simulink model "Projet_Controle_Trajectoire_drone"  (R2024a)
settings: Solver=ode4  StartTime=0.0  StopTime=Tfinsim  FixedStep=Tech  RelTol=1e-3
values from neighbouring files (symbols this model uses):
  A = [Axx, 0, 0; 0, Ayy, 0; 0, 0, Azz]    [Project_Drone_run.m]    (also in Projet_Controle_Trajectoire_drone_run.m)
  b = 7.5*10^-7    (= 7.5e-07)    [Project_Drone_run.m]    (also in Projet_Controle_Trajectoire_drone_run.m)
  Biais = 0.024    [Project_Drone_run.m]    (also in Projet_Controle_Trajectoire_drone_run.m)
  Bruit = 0.002    [Project_Drone_run.m]    (also in Projet_Controle_Trajectoire_drone_run.m)
  g = 9.81    [Project_Drone_run.m]    (also in Projet_Controle_Trajectoire_drone_run.m)
  I = [Ixx, Ixy, Ixz; Iyx, Iyy, Iyz; Izx, Izy, Izz]    [Project_Drone_run.m]    (also in Projet_Controle_Trajectoire_drone_run.m)
  I_M = 6.24*10^-6    (= 6.24e-06)    [Project_Drone_run.m]    (also in Projet_Controle_Trajectoire_drone_run.m)
  Iinv = I^-1    [Project_Drone_run.m]    (also in Projet_Controle_Trajectoire_drone_run.m)
  Ixx = 0.01    [Project_Drone_run.m]    (also in Projet_Controle_Trajectoire_drone_run.m)
  Iyy = 0.011    [Project_Drone_run.m]    (also in Projet_Controle_Trajectoire_drone_run.m)
  Izz = 0.019    [Project_Drone_run.m]    (also in Projet_Controle_Trajectoire_drone_run.m)
  k = 3.13E-5    (= 3.13e-05)    [Project_Drone_run.m]    (also in Projet_Controle_Trajectoire_drone_run.m)
  KdPhi = 30    [Project_Drone_run.m]    (also in Projet_Controle_Trajectoire_drone_run.m)
  KdPsi = 30    [Project_Drone_run.m]    (also in Projet_Controle_Trajectoire_drone_run.m)
  KdTheta = 30    [Project_Drone_run.m]    (also in Projet_Controle_Trajectoire_drone_run.m)
  KdU = 0    [Project_Drone_run.m]    (also in Projet_Controle_Trajectoire_drone_run.m)
  KdV = 0    [Project_Drone_run.m]    (also in Projet_Controle_Trajectoire_drone_run.m)
  KdZ = 8    [Project_Drone_run.m]    (also in Projet_Controle_Trajectoire_drone_run.m)
  KiPhi = 10    [Project_Drone_run.m]    (also in Projet_Controle_Trajectoire_drone_run.m)
  KiPsi = 10    [Project_Drone_run.m]    (also in Projet_Controle_Trajectoire_drone_run.m)
  KiTheta = 10    [Project_Drone_run.m]    (also in Projet_Controle_Trajectoire_drone_run.m)
  KiU = 0.2    [Project_Drone_run.m]    (also in Projet_Controle_Trajectoire_drone_run.m)
  KiV = 0.2    [Project_Drone_run.m]    (also in Projet_Controle_Trajectoire_drone_run.m)
  KiZ = 0    [Project_Drone_run.m]    (also in Projet_Controle_Trajectoire_drone_run.m)
  KpPhi = 190    [Project_Drone_run.m]    (also in Projet_Controle_Trajectoire_drone_run.m)
  KpPsi = 190    [Project_Drone_run.m]    (also in Projet_Controle_Trajectoire_drone_run.m)
  KpTheta = 190    [Project_Drone_run.m]    (also in Projet_Controle_Trajectoire_drone_run.m)
  KpU = 0.6    [Project_Drone_run.m]    (also in Projet_Controle_Trajectoire_drone_run.m)
  KpV = 0.6    [Project_Drone_run.m]    (also in Projet_Controle_Trajectoire_drone_run.m)
  KpZ = 20    [Project_Drone_run.m]    (also in Projet_Controle_Trajectoire_drone_run.m)
  l = 0.23    [Project_Drone_run.m]    (also in Projet_Controle_Trajectoire_drone_run.m)
  m = 1.232    [Project_Drone_run.m]    (also in Projet_Controle_Trajectoire_drone_run.m)
  Psic = 0    [Project_Drone_run.m]    (also in Projet_Controle_Trajectoire_drone_run.m)
  R = [sqrt(2)/2, sqrt(2)/2, 0; -sqrt(2)/2, sqrt(2)/2, 0; 0, 0, 1]    [Project_Drone_run.m]    (also in Projet_Controle_Trajectoire_drone_run.m)
  retard = 0.001    [Project_Drone_run.m]    (also in Projet_Controle_Trajectoire_drone_run.m)
  Rt = transpose(R)    [Project_Drone_run.m]    (also in Projet_Controle_Trajectoire_drone_run.m)
  Xc = 0    [Project_Drone_run.m]    (also in Projet_Controle_Trajectoire_drone_run.m)
  Yc = 0    [Project_Drone_run.m]    (also in Projet_Controle_Trajectoire_drone_run.m)
  Zc = 1.5    [Project_Drone_run.m]    (also in Projet_Controle_Trajectoire_drone_run.m)
libraries: simulink x6, matrix_library x3, visionfilter x1
settings Model: Creator=mbeauchet  LastModifiedBy=caste

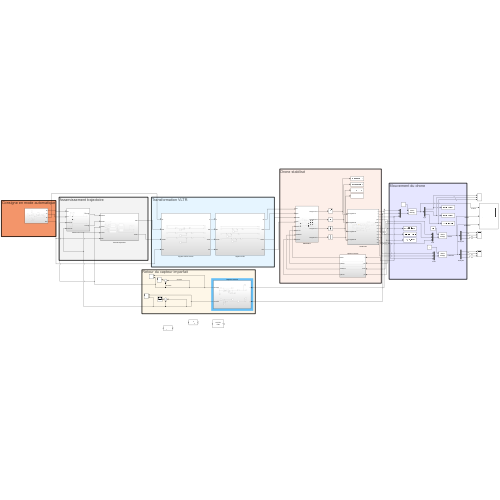
[thumbnail: Simulink's stored preview of the top-level diagram]
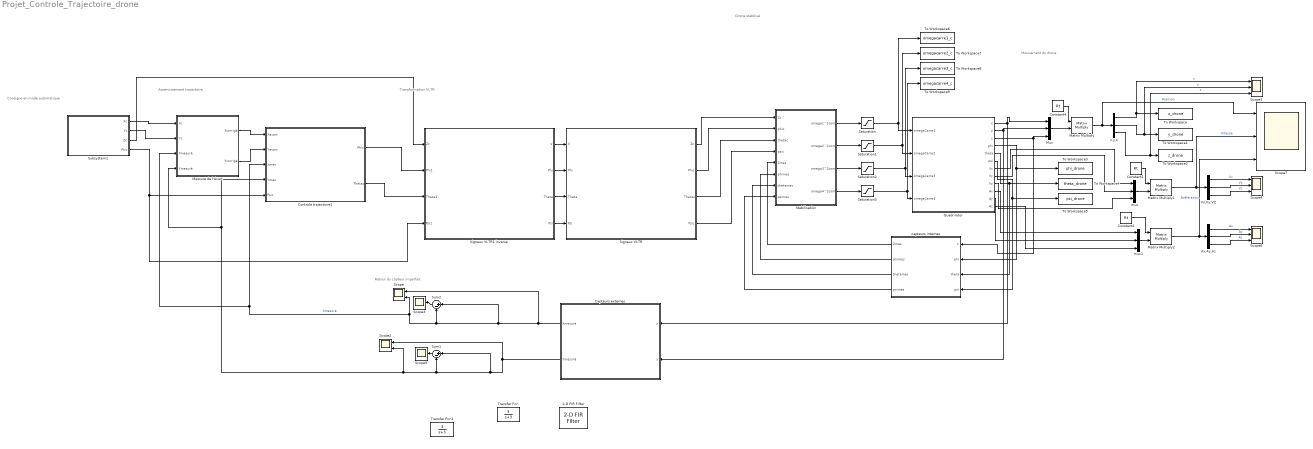
== system Projet_Controle_Trajectoire_drone ==
  note: Retour du capteur imparfait
  note: Consigne en mode automatique
  note: Asservissement trajectoire
  note: Transformation VLTR
  note: Drone stabilisé
  note: Mouvement du drone
  2-D FIR Filter : visionfilter/2-D FIR Filter  separable=off  filtSrc=Specify via dialog  filterMtrx=[0.9]  verticalFilter=[4 0]  horizontalFilter=[4 0]  outSize=Full  padType=Constant  padSrc=Specify via dialog  padVal=0  method=Convolution  firstCoeffMode=Specify word length  firstCoeffWordLength=16  firstCoeffFracLength=14  firstCoeffSignedness=Signed  firstCoeffLastDataTypeStr=fixdt(1,16)  outputSignedness=Auto  accumLastDataTypeStr=Inherit: Same as product output  prodOutputMode=Binary point scaling  prodOutputWordLength=32  prodOutputFracLength=10  prodOutputLastDataTypeStr=fixdt([],32,10)  roundingMode=Floor  overflowMode=off  firstCoeffDataTypeStr=fixdt(1,16)  firstCoeffMin=[]  firstCoeffMax=[]  prodOutputDataTypeStr=fixdt([],32,10)  accumDataTypeStr=Inherit: Same as product output  outputMin=[]  outputMax=[]
  Ax,Ay,Az : Demux  Outputs=3
  Capteurs externes : Subsystem
  Constant1 : Constant  Value=Rt
  Constant2 : Constant  Value=Rt
  Constant4 : Constant  Value=Rt
  Controle trajectoire1 : Subsystem
  Matrix Multiply : Product  Multiplication=Matrix(*)
  Matrix Multiply1 : Product  Multiplication=Matrix(*)
  Matrix Multiply2 : Product  Multiplication=Matrix(*)
  Messure de l'écart : Subsystem
  Mux : Mux  Inputs=3
  Quadrirotor : Subsystem
  Saturation{,1..3} (4 alike) : Saturate  UpperLimit=(10464*(2*pi)/60)^2  LowerLimit=-(10464*2*pi/60)^2
  Scope : Scope  NumInputPorts=2
  Scope{1,4,6..7} (4 alike) : Scope  NumInputPorts=3
  Scope2 : Scope  NumInputPorts=2
  Scope3 : Scope
  Scope5 : Scope
  Signaux VLTR : Subsystem
  Signaux VLTR1 inverse : Subsystem
  Stabilisation : Subsystem
  Subsystem1 : Subsystem
  Sum1 : Sum  Inputs=|+-
  Sum2 : Sum  Inputs=|+-
  To Workspace : ToWorkspace  VariableName=x_drone  SaveFormat=Structure With Time  SampleTime=-1
  To Workspace1 : ToWorkspace  VariableName=y_drone  SaveFormat=Structure With Time  SampleTime=-1
  To Workspace2 : ToWorkspace  VariableName=z_drone  SaveFormat=Structure With Time  SampleTime=-1
  To Workspace3 : ToWorkspace  VariableName=phi_drone  SaveFormat=Structure With Time  SampleTime=-1
  To Workspace4 : ToWorkspace  VariableName=theta_drone  SaveFormat=Structure With Time  SampleTime=-1
  To Workspace5 : ToWorkspace  VariableName=psi_drone  SaveFormat=Structure With Time  SampleTime=-1
  To Workspace6 : ToWorkspace  VariableName=omegacarre1_c  SaveFormat=Structure With Time  SampleTime=-1
  To Workspace7 : ToWorkspace  VariableName=omegacarre2_c  SaveFormat=Structure With Time  SampleTime=-1
  To Workspace8 : ToWorkspace  VariableName=omegacarre3_c  SaveFormat=Structure With Time  SampleTime=-1
  To Workspace9 : ToWorkspace  VariableName=omegacarre4_c  SaveFormat=Structure With Time  SampleTime=-1
  Transfer Fcn : TransferFcn  Numerator=[3]  Denominator=[1 3]
  Transfer Fcn1 : TransferFcn  Numerator=[3]  Denominator=[1 3]
  Vx,Vy,VZ : Demux  Outputs=3
  capteurs internes : Subsystem
  mux : Mux  Inputs=3
  mux1 : Mux  Inputs=3
  x,y,z : Demux  Outputs=3
  wires:
  Quadrirotor/1(x) -> Mux/1, Capteurs externes/1(x)
  Subsystem1/2(Yc) -> Messure de l'écart/2(Yc)
  Signaux VLTR1 inverse/3(Theta) -> Signaux VLTR/3(Theta)
  x,y,z/2 -> To Workspace1/1, Scope1/2  "y"
  Signaux VLTR/3(Thetac) -> Stabilisation/3(thetac)
  Quadrirotor/2(y) -> Capteurs externes/2(y), Mux/2
  x,y,z/1 -> To Workspace/1, Scope1/1  "x"
  Signaux VLTR/4(Psic) -> Stabilisation/4(psic)
  Matrix Multiply/1 -> Scope7/1, x,y,z/1  "Position"
  Controle trajectoire1/1(Phic) -> Signaux VLTR1 inverse/2(Phi1)
  Constant4/1 -> Matrix Multiply/1
  x,y,z/3 -> To Workspace2/1, Scope1/3  "z"
  capteurs internes/2(phimes) -> Stabilisation/6(phimes)
  Subsystem1/1(Xc) -> Messure de l'écart/1(Xc)
  Subsystem1/3(Zc) -> Signaux VLTR1 inverse/1(Zc)
  Quadrirotor/5(theta) -> capteurs internes/3(theta), To Workspace4/1
  Messure de l'écart/2(Ycorrigé) -> Controle trajectoire1/2(Yecart)
  Signaux VLTR/2(Phic) -> Stabilisation/2(phic)
  Signaux VLTR1 inverse/2(Phi) -> Signaux VLTR/2(Phi)
  Signaux VLTR1 inverse/4(Psi) -> Signaux VLTR/4(Psi)
  Saturation1/1 -> Quadrirotor/2(omegaCarre2), To Workspace7/1
  Quadrirotor/6(psi) -> capteurs internes/4(psi), To Workspace5/1
  Saturation3/1 -> Quadrirotor/4(omegaCarre4), To Workspace9/1
  Mux/1 -> Matrix Multiply/2
  capteurs internes/1(Zmes) -> Stabilisation/5(Zmes)
  Saturation/1 -> Quadrirotor/1(omegaCarre1), To Workspace6/1
  Saturation2/1 -> Quadrirotor/3(omegaCarre3), To Workspace8/1
  Messure de l'écart/1(Xcorrigé) -> Controle trajectoire1/1(Xecart)
  capteurs internes/4(psimes) -> Stabilisation/8(psimes)
  Quadrirotor/4(phi) -> capteurs internes/2(phi), To Workspace3/1
  Stabilisation/4(omega4^2com) -> Saturation3/1
  Quadrirotor/3(z) -> capteurs internes/1(z), Mux/3
  Subsystem1/4(Psic) -> Signaux VLTR1 inverse/4(Psi1), Controle trajectoire1/5(Psic)
  Controle trajectoire1/2(Thetac) -> Signaux VLTR1 inverse/3(Theta1)
  Stabilisation/1(omega1^2com) -> Saturation/1
  Stabilisation/3(omega3^2com) -> Saturation2/1
  capteurs internes/3(thetames) -> Stabilisation/7(thetames)
  Stabilisation/2(omega2^2com) -> Saturation1/1
  Sum1/1 -> Scope5/1
  Sum2/1 -> Scope3/1
  Signaux VLTR1 inverse/1(V) -> Signaux VLTR/1(V)
  Signaux VLTR/1(Zc) -> Stabilisation/1(Zc)
  mux/1 -> Matrix Multiply1/2
  Quadrirotor/7(Vx) -> mux/1
  Quadrirotor/8(Vy) -> mux/2
  Constant1/1 -> Matrix Multiply1/1
  Quadrirotor/9(Vz) -> mux/3
  mux1/1 -> Matrix Multiply2/2
  Quadrirotor/10(Ax) -> mux1/1
  Quadrirotor/11(Ay) -> mux1/2
  Constant2/1 -> Matrix Multiply2/1
  Quadrirotor/12(Az) -> mux1/3
  Vx,Vy,VZ/1 -> Scope4/1  "Vx"
  Vx,Vy,VZ/2 -> Scope4/2  "Vy"
  Vx,Vy,VZ/3 -> Scope4/3  "Vz"
  Ax,Ay,Az/1 -> Scope6/1  "Ax"
  Ax,Ay,Az/2 -> Scope6/2  "Ay"
  Ax,Ay,Az/3 -> Scope6/3  "Az"
  Matrix Multiply2/1 -> Scope7/3, Ax,Ay,Az/1  "Acélération"
  Matrix Multiply1/1 -> Scope7/2, Vx,Vy,VZ/1  "Vitesse"
  Capteurs externes/1(Xmesuré) -> Sum2/2, Messure de l'écart/3(Xmesuré), Controle trajectoire1/3(Xmes), Scope/2, Sum2/1, Scope/1  "Xmesuré"
  Capteurs externes/2(Ymesuré) -> Sum1/2, Scope2/2, Controle trajectoire1/4(Ymes), Messure de l'écart/4(Ymesuré), Sum1/1, Scope2/1

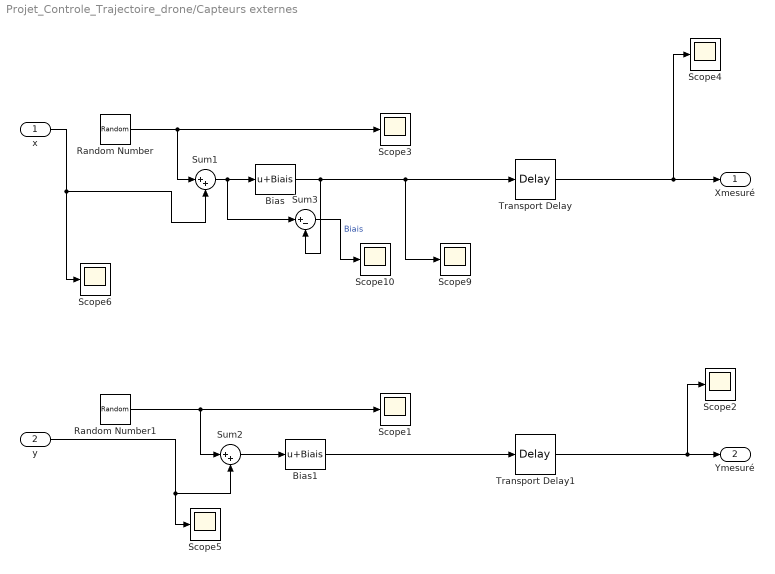
== system Projet_Controle_Trajectoire_drone/Capteurs externes ==
  x : Inport
  y : Inport  Port=2
  Bias : Bias  Bias=Biais  SaturateOnIntegerOverflow=off
  Bias1 : Bias  Bias=Biais  SaturateOnIntegerOverflow=off
  Random Number : RandomNumber  Variance=Bruit  SampleTime=0.07
  Random Number1 : RandomNumber  Variance=Bruit  SampleTime=0.07
  Scope{1..6,9..10} (8 alike) : Scope
  Sum1 : Sum  Inputs=|++
  Sum2 : Sum  Inputs=|++
  Sum3 : Sum  Inputs=|+-
  Transport Delay : TransportDelay  DelayTime=retard
  Transport Delay1 : TransportDelay  DelayTime=retard
  Xmesuré : Outport
  Ymesuré : Outport  Port=2
  wires:
  Sum2/1 -> Bias1/1
  x/1 -> Scope6/1, Sum1/2
  Random Number1/1 -> Sum2/1, Scope1/1
  Random Number/1 -> Scope3/1, Sum1/1
  y/1 -> Scope5/1, Sum2/2
  Sum1/1 -> Sum3/1, Bias/1
  Bias/1 -> Sum3/2, Transport Delay/1, Scope9/1
  Bias1/1 -> Transport Delay1/1
  Transport Delay/1 -> Xmesuré/1, Scope4/1
  Transport Delay1/1 -> Ymesuré/1, Scope2/1
  Sum3/1 -> Scope10/1  "Biais"

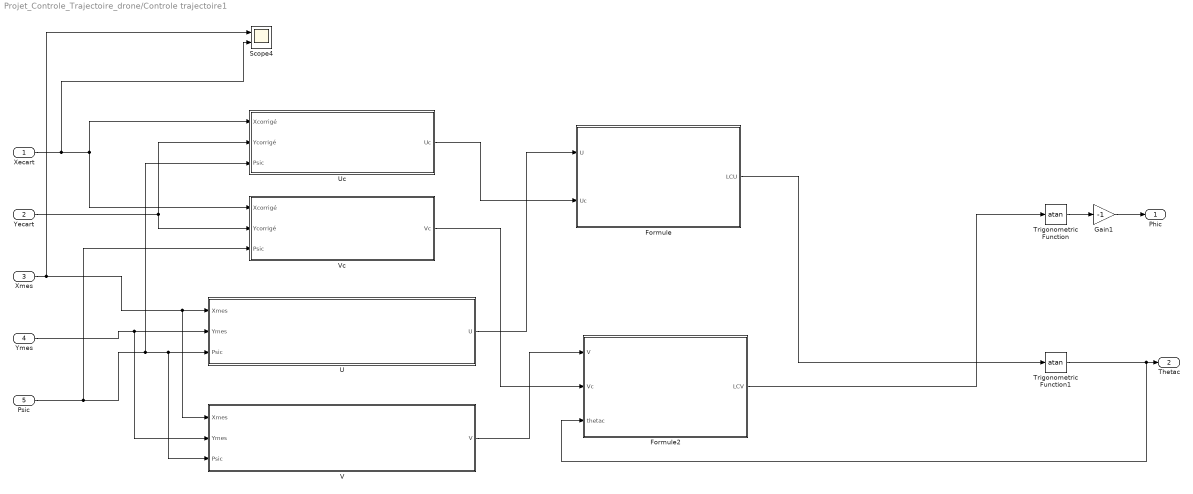
== system Projet_Controle_Trajectoire_drone/Controle trajectoire1 ==
  Xecart : Inport
  Yecart : Inport  Port=2
  Xmes : Inport  Port=3
  Ymes : Inport  Port=4
  Psic : Inport  Port=5
  Formule : Subsystem
  Formule2 : Subsystem
  Gain1 : Gain  Gain=-1
  Scope4 : Scope  NumInputPorts=2
  Trigonometric Function : Trigonometry  Operator=atan
  Trigonometric Function1 : Trigonometry  Operator=atan
  U : Subsystem
  Uc : Subsystem
  V : Subsystem
  Vc : Subsystem
  Phic : Outport
  Thetac : Outport  Port=2
  wires:
  Psic/1 -> Vc/3(Psic), Uc/3(Psic), V/3(Psic), U/3(Psic)
  Ymes/1 -> V/2(Ymes), U/2(Ymes)
  Xmes/1 -> Scope4/1, V/1(Xmes), U/1(Xmes)
  Yecart/1 -> Vc/2(Ycorrigé), Uc/2(Ycorrigé)
  Trigonometric Function1/1 -> Formule2/3(thetac), Thetac/1
  U/1(U) -> Formule/1(U)
  Uc/1(Uc) -> Formule/2(Uc)
  Formule/1(LCU) -> Trigonometric Function1/1
  Formule2/1(LCV) -> Trigonometric Function/1
  V/1(V) -> Formule2/1(V)
  Vc/1(Vc) -> Formule2/2(Vc)
  Trigonometric Function/1 -> Gain1/1
  Gain1/1 -> Phic/1
  Xecart/1 -> Scope4/2, Vc/1(Xcorrigé), Uc/1(Xcorrigé)

== system Projet_Controle_Trajectoire_drone/Messure de l'écart ==
  Xc : Inport
  Yc : Inport  Port=2
  Xmesuré : Inport  Port=3
  Ymesuré : Inport  Port=4
  Scope{,1..3} (4 alike) : Scope
  Sum4 : Sum  Inputs=|+-
  Sum5 : Sum  Inputs=|+-
  Xcorrigé : Outport
  Ycorrigé : Outport  Port=2
  wires:
  Sum5/1 -> Scope1/1, Xcorrigé/1, Scope/1
  Xc/1 -> Scope2/1, Sum5/1
  Xmesuré/1 -> Sum5/2, Scope3/1
  Yc/1 -> Sum4/1
  Ymesuré/1 -> Sum4/2
  Sum4/1 -> Ycorrigé/1

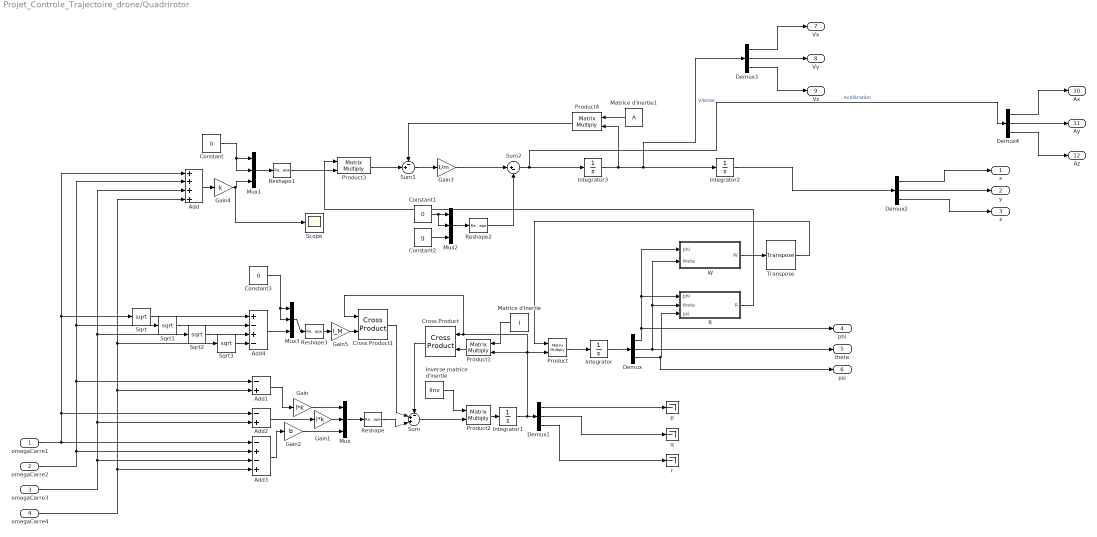
== system Projet_Controle_Trajectoire_drone/Quadrirotor ==
  omegaCarre1 : Inport  PortDimensions=1
  omegaCarre2 : Inport  Port=2  PortDimensions=1
  omegaCarre3 : Inport  Port=3  PortDimensions=1
  omegaCarre4 : Inport  Port=4  PortDimensions=1
  Add : Sum  Inputs=++++
  Add1 : Sum  Inputs=-+
  Add2 : Sum  Inputs=-+
  Add3 : Sum  Inputs=-+-+
  Add4 : Sum  Inputs=+-+-
  Constant : Constant  Value=0
  Constant1 : Constant  Value=0
  Constant2 : Constant  Value=g
  Constant3 : Constant  Value=0
  Cross Product : matrix_library/Cross Product
  Cross Product1 : matrix_library/Cross Product
  Demux{,1..4} (5 alike) : Demux  Outputs=3
  Gain : Gain  Gain=l*k
  Gain1 : Gain  Gain=l*k
  Gain2 : Gain  Gain=b
  Gain3 : Gain  Gain=1/m
  Gain4 : Gain  Gain=k
  Gain5 : Gain  Gain=I_M
  Integrator{,1..3} (4 alike) : Integrator
  Inverse matrice d'inertie : Constant  Value=Iinv
  Matrice d'inertie : Constant  Value=I
  Matrice d'inertie1 : Constant  Value=A
  Mux{,1..3} (4 alike) : Mux  Inputs=3
  Product{,1..4} (5 alike) : Product  Multiplication=Matrix(*)
  R : Subsystem
  Reshape{,1..3} (4 alike) : Reshape  OutputDimensionality=Column vector (2-D)
  Scope : Scope
  Sqrt{,1..3} (4 alike) : Sqrt
  Sum : Sum  Inputs=-++|
  Sum1 : Sum  Inputs=-+|
  Sum2 : Sum  Inputs=|+-
  Transpose : matrix_library/Transpose
  W : Subsystem
  p : Terminator
  q : Terminator
  r : Terminator
  x : Outport
  y : Outport  Port=2
  z : Outport  Port=3
  phi : Outport  Port=4
  theta : Outport  Port=5
  psi : Outport  Port=6
  Vx : Outport  Port=7
  Vy : Outport  Port=8
  Vz : Outport  Port=9
  Ax : Outport  Port=10
  Ay : Outport  Port=11
  Az : Outport  Port=12
  wires:
  Gain5/1 -> Cross Product1/2
  Sqrt2/1 -> Add4/3
  Mux3/1 -> Reshape3/1
  Demux2/3 -> z/1
  Reshape3/1 -> Gain5/1
  Constant3/1 -> Mux3/2, Mux3/1
  Transpose/1 -> Product/1
  Mux1/1 -> Reshape1/1
  Product1/1 -> Cross Product/2
  Demux1/2 -> q/1
  Sqrt3/1 -> Add4/4
  Demux1/3 -> r/1
  omegaCarre2/1 -> Add3/2, Add1/1, Sqrt1/1, Add/2
  Constant/1 -> Mux1/2, Mux1/1
  Constant2/1 -> Mux2/3
  Demux/2 -> theta/1, R/2(theta), W/2(theta)
  Cross Product1/1 -> Sum/2
  Demux1/1 -> p/1
  Add/1 -> Gain4/1
  Sqrt/1 -> Add4/1
  Mux2/1 -> Reshape2/1
  Demux/1 -> phi/1, R/1(phi), W/1(phi)
  Sum1/1 -> Gain3/1
  Add1/1 -> Gain/1
  Integrator/1 -> Demux/1
  Matrice d'inertie1/1 -> Product4/1
  Constant1/1 -> Mux2/2, Mux2/1
  Add3/1 -> Gain2/1
  Inverse matrice d'inertie/1 -> Product2/1
  Reshape/1 -> Sum/3
  omegaCarre4/1 -> Add3/4, Add1/2, Sqrt3/1, Add/4
  omegaCarre3/1 -> Add3/3, Add2/2, Add/3, Sqrt2/1
  Add4/1 -> Mux3/3
  Gain2/1 -> Mux/3
  Product2/1 -> Integrator1/1
  Add2/1 -> Gain1/1
  Demux2/1 -> x/1
  Gain1/1 -> Mux/2
  Integrator1/1 -> Product1/2, Cross Product1/1, Cross Product/1, Product/2, Demux1/1
  Sqrt1/1 -> Add4/2
  Product/1 -> Integrator/1
  Gain4/1 -> Scope/1, Mux1/3
  Reshape2/1 -> Sum2/2
  W/1(W) -> Transpose/1
  Sum/1 -> Product2/2
  Gain/1 -> Mux/1
  Cross Product/1 -> Sum/1
  Gain3/1 -> Sum2/1
  Product4/1 -> Sum1/1
  R/1(R) -> Product3/1
  Matrice d'inertie/1 -> Product1/1
  Product3/1 -> Sum1/2
  Demux2/2 -> y/1
  Mux/1 -> Reshape/1
  Reshape1/1 -> Product3/2
  omegaCarre1/1 -> Sqrt/1, Add/1, Add2/1, Add3/1
  Demux/3 -> R/3(psi), psi/1
  Demux3/1 -> Vx/1
  Demux3/2 -> Vy/1
  Demux3/3 -> Vz/1
  Demux4/3 -> Az/1
  Demux4/2 -> Ay/1
  Demux4/1 -> Ax/1
  Integrator2/1 -> Demux2/1
  Integrator3/1 -> Integrator2/1, Demux3/1, Product4/2  "Vitesse"
  Sum2/1 -> Integrator3/1, Demux4/1  "Acélération"

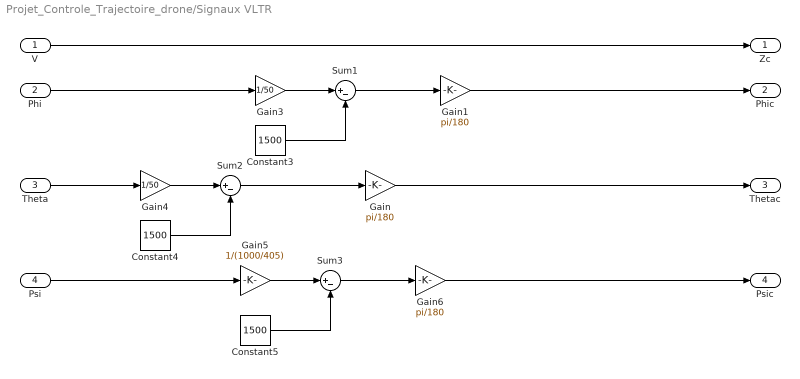
== system Projet_Controle_Trajectoire_drone/Signaux VLTR ==
  V : Inport
  Phi : Inport  Port=2
  Theta : Inport  Port=3
  Psi : Inport  Port=4
  Constant3 : Constant  Value=1500
  Constant4 : Constant  Value=1500
  Constant5 : Constant  Value=1500
  Gain : Gain  Gain=pi/180
  Gain1 : Gain  Gain=pi/180
  Gain3 : Gain  Gain=1/50
  Gain4 : Gain  Gain=1/50
  Gain5 : Gain  Gain=1/(1000/405)
  Gain6 : Gain  Gain=pi/180
  Sum1 : Sum  Inputs=|+-
  Sum2 : Sum  Inputs=|+-
  Sum3 : Sum  Inputs=|+-
  Zc : Outport
  Phic : Outport  Port=2
  Thetac : Outport  Port=3
  Psic : Outport  Port=4
  wires:
  Constant3/1 -> Sum1/2
  Gain4/1 -> Sum2/1
  Sum1/1 -> Gain1/1
  Constant5/1 -> Sum3/2
  Sum2/1 -> Gain/1
  Gain5/1 -> Sum3/1
  Constant4/1 -> Sum2/2
  Sum3/1 -> Gain6/1
  Gain3/1 -> Sum1/1
  Psi/1 -> Gain5/1
  Gain1/1 -> Phic/1
  Gain/1 -> Thetac/1
  Gain6/1 -> Psic/1
  Phi/1 -> Gain3/1
  Theta/1 -> Gain4/1
  V/1 -> Zc/1

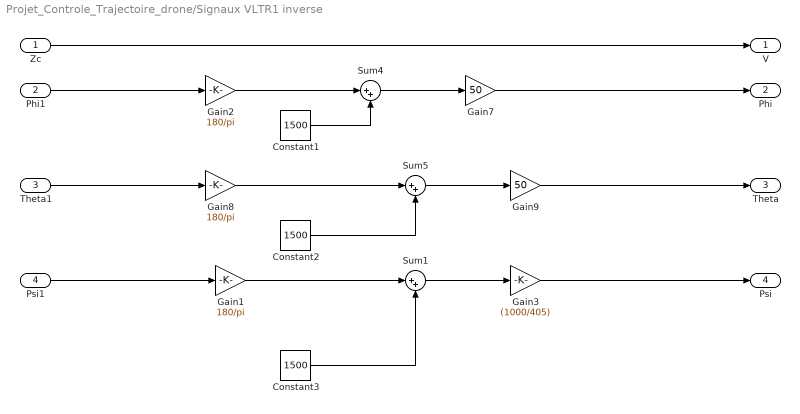
== system Projet_Controle_Trajectoire_drone/Signaux VLTR1 inverse ==
  Zc : Inport
  Phi1 : Inport  Port=2
  Theta1 : Inport  Port=3
  Psi1 : Inport  Port=4
  Constant1 : Constant  Value=1500
  Constant2 : Constant  Value=1500
  Constant3 : Constant  Value=1500
  Gain1 : Gain  Gain=180/pi
  Gain2 : Gain  Gain=180/pi
  Gain3 : Gain  Gain=(1000/405)
  Gain7 : Gain  Gain=50
  Gain8 : Gain  Gain=180/pi
  Gain9 : Gain  Gain=50
  Sum1 : Sum  Inputs=|++
  Sum4 : Sum  Inputs=|++
  Sum5 : Sum  Inputs=|++
  V : Outport
  Phi : Outport  Port=2
  Theta : Outport  Port=3
  Psi : Outport  Port=4
  wires:
  Constant1/1 -> Sum4/2
  Gain2/1 -> Sum4/1
  Sum4/1 -> Gain7/1
  Gain8/1 -> Sum5/1
  Sum5/1 -> Gain9/1
  Constant2/1 -> Sum5/2
  Constant3/1 -> Sum1/2
  Gain1/1 -> Sum1/1
  Sum1/1 -> Gain3/1
  Phi1/1 -> Gain2/1
  Gain7/1 -> Phi/1
  Theta1/1 -> Gain8/1
  Gain9/1 -> Theta/1
  Psi1/1 -> Gain1/1
  Gain3/1 -> Psi/1
  Zc/1 -> V/1

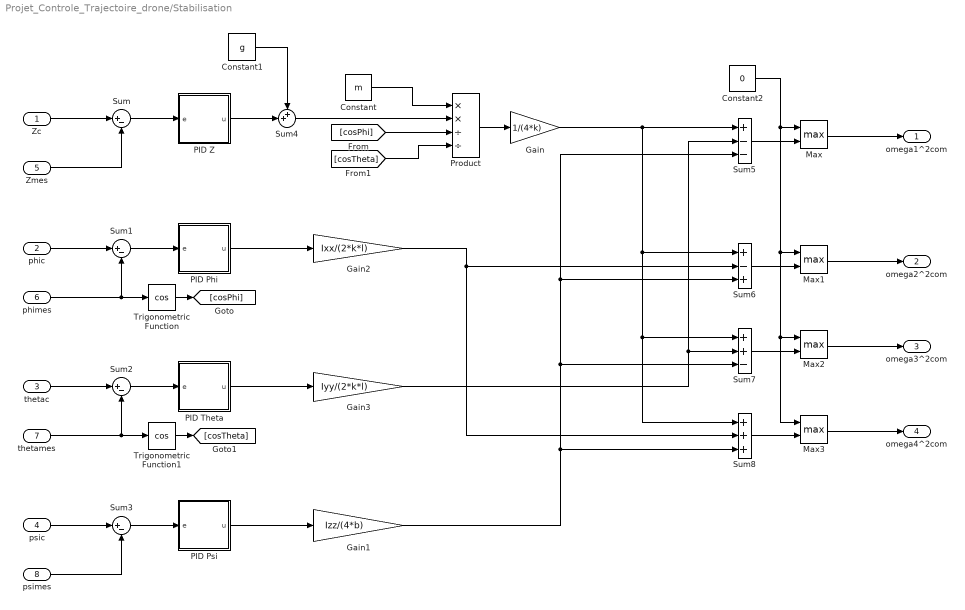
== system Projet_Controle_Trajectoire_drone/Stabilisation ==
  Zc : Inport
  phic : Inport  Port=2
  thetac : Inport  Port=3
  psic : Inport  Port=4
  Zmes : Inport  Port=5
  phimes : Inport  Port=6
  thetames : Inport  Port=7
  psimes : Inport  Port=8
  Constant : Constant  Value=m
  Constant1 : Constant  Value=g
  Constant2 : Constant  Value=0
  Gain : Gain  Gain=1/(4*k)
  Gain1 : Gain  Gain=Izz/(4*b)
  Gain2 : Gain  Gain=Ixx/(2*k*l)
  Gain3 : Gain  Gain=Iyy/(2*k*l)
  Max{,1..3} (4 alike) : MinMax  Function=max  Inputs=2
  PID Phi : Subsystem
  PID Psi : Subsystem
  PID Theta : Subsystem
  PID Z : Subsystem
  Product : Product  Inputs=**//
  Sum{,1..3} (4 alike) : Sum  Inputs=|+-
  Sum4 : Sum  Inputs=++|
  Sum5 : Sum  Inputs=+--
  Sum6 : Sum  Inputs=+-+
  Sum7 : Sum  Inputs=++-
  Sum8 : Sum  Inputs=+++
  Trigonometric Function : Trigonometry  Operator=cos
  Trigonometric Function1 : Trigonometry  Operator=cos
  omega1^2com : Outport
  omega2^2com : Outport  Port=2
  omega3^2com : Outport  Port=3
  omega4^2com : Outport  Port=4
  wires:
  Max2/1 -> omega3^2com/1
  Max/1 -> omega1^2com/1
  Sum6/1 -> Max1/2
  Gain2/1 -> Sum8/2, Sum6/2
  Max1/1 -> omega2^2com/1
  PID Theta/1(u) -> Gain3/1
  Sum4/1 -> Product/2
  Trigonometric Function/1 -> [cosPhi]
  Max3/1 -> omega4^2com/1
  phimes/1 -> Trigonometric Function/1, Sum1/2
  Sum5/1 -> Max/2
  Sum8/1 -> Max3/2
  Constant2/1 -> Max3/1, Max2/1, Max1/1, Max/1
  Gain1/1 -> Sum8/3, Sum7/3, Sum6/3, Sum5/3
  psimes/1 -> Sum3/2
  PID Psi/1(u) -> Gain1/1
  PID Phi/1(u) -> Gain2/1
  Constant1/1 -> Sum4/1
  [cosTheta] -> Product/4
  Constant/1 -> Product/1
  Gain3/1 -> Sum7/2, Sum5/2
  PID Z/1(u) -> Sum4/2
  [cosPhi] -> Product/3
  Gain/1 -> Sum8/1, Sum7/1, Sum6/1, Sum5/1
  Zmes/1 -> Sum/2
  Trigonometric Function1/1 -> [cosTheta]
  psic/1 -> Sum3/1
  Product/1 -> Gain/1
  Sum/1 -> PID Z/1(e)
  Sum7/1 -> Max2/2
  thetames/1 -> Sum2/2, Trigonometric Function1/1
  Zc/1 -> Sum/1
  Sum1/1 -> PID Phi/1(e)
  Sum2/1 -> PID Theta/1(e)
  Sum3/1 -> PID Psi/1(e)
  thetac/1 -> Sum2/1
  phic/1 -> Sum1/1

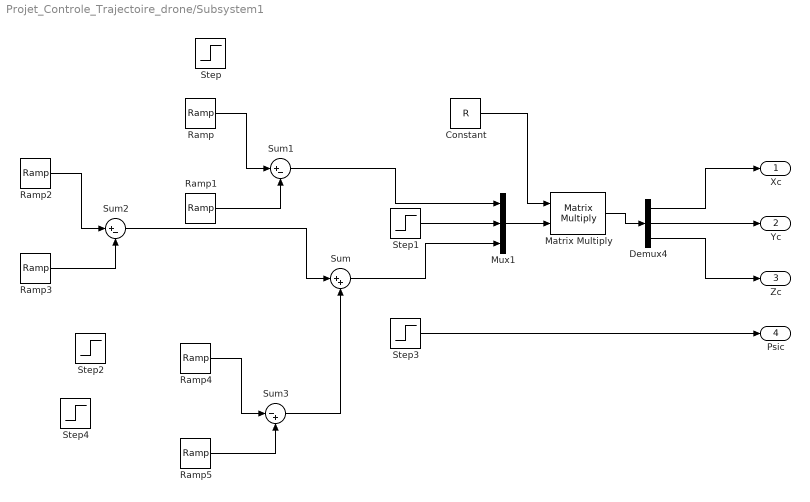
== system Projet_Controle_Trajectoire_drone/Subsystem1 ==
  Constant : Constant  Value=R
  Demux4 : Demux  Outputs=3
  Matrix Multiply : Product  Multiplication=Matrix(*)
  Mux1 : Mux  Inputs=3
  Ramp : simulink/Sources/Ramp  slope=0.5  start=12  InitialOutput=0
  Ramp1 : simulink/Sources/Ramp  slope=0.5  start=42  InitialOutput=0
  Ramp2 : simulink/Sources/Ramp  slope=0.5  start=0  InitialOutput=0
  Ramp3 : simulink/Sources/Ramp  slope=0.5  start=3  InitialOutput=0
  Ramp4 : simulink/Sources/Ramp  slope=0.5  start=50  InitialOutput=0
  Ramp5 : simulink/Sources/Ramp  slope=0.5  start=53  InitialOutput=0
  Step : Step  Time=12  After=Xc  SampleTime=0
  Step1 : Step  After=Yc  SampleTime=0
  Step2 : Step  Time=0  After=Zc  SampleTime=0
  Step3 : Step  Time=0  After=Psic  SampleTime=0
  Step4 : Step  Time=50  After=-Zc  SampleTime=0
  Sum : Sum  Inputs=|++
  Sum1 : Sum  Inputs=|+-
  Sum2 : Sum  Inputs=|+-
  Sum3 : Sum  Inputs=|-+
  Xc : Outport
  Yc : Outport  Port=2
  Zc : Outport  Port=3
  Psic : Outport  Port=4
  wires:
  Step3/1 -> Psic/1
  Ramp/1 -> Sum1/1
  Constant/1 -> Matrix Multiply/1
  Step1/1 -> Mux1/2
  Mux1/1 -> Matrix Multiply/2
  Matrix Multiply/1 -> Demux4/1
  Demux4/1 -> Xc/1
  Demux4/2 -> Yc/1
  Demux4/3 -> Zc/1
  Sum/1 -> Mux1/3
  Ramp1/1 -> Sum1/2
  Sum1/1 -> Mux1/1
  Ramp3/1 -> Sum2/2
  Sum2/1 -> Sum/1
  Ramp2/1 -> Sum2/1
  Ramp4/1 -> Sum3/1
  Ramp5/1 -> Sum3/2
  Sum3/1 -> Sum/2

== system Projet_Controle_Trajectoire_drone/capteurs internes ==
  z : Inport
  phi : Inport  Port=2
  theta : Inport  Port=3
  psi : Inport  Port=4
  Zmes : Outport
  phimes : Outport  Port=2
  thetames : Outport  Port=3
  psimes : Outport  Port=4
  wires:
  psi/1 -> psimes/1
  theta/1 -> thetames/1
  phi/1 -> phimes/1
  z/1 -> Zmes/1

== system Projet_Controle_Trajectoire_drone/Controle trajectoire1/Formule ==
  U : Inport
  Uc : Inport  Port=2
  Add1 : Sum  Inputs=+-
  Derivative : Derivative
  Gain : Gain  Gain=KpU
  Gain1 : Gain  Gain=KiU
  Gain2 : Gain  Gain=KdU
  Sum : Sum  Inputs=+|+-
  LCU : Outport
  wires:
  Sum/1 -> LCU/1
  Gain/1 -> Sum/2
  Gain1/1 -> Sum/1
  Gain2/1 -> Derivative/1
  Derivative/1 -> Sum/3
  U/1 -> Add1/2, Gain2/1
  Uc/1 -> Gain1/1, Add1/1
  Add1/1 -> Gain/1

== system Projet_Controle_Trajectoire_drone/Controle trajectoire1/Formule2 ==
  V : Inport
  Vc : Inport  Port=2
  thetac : Inport  Port=3
  Add1 : Sum  Inputs=+-
  Derivative : Derivative
  Gain : Gain  Gain=KpV
  Gain1 : Gain  Gain=KiV
  Gain2 : Gain  Gain=KdV
  Product : Product
  Sum : Sum  Inputs=+|+-
  Trigonometric Function1 : Trigonometry  Operator=cos
  LCV : Outport
  wires:
  Gain/1 -> Sum/2
  Gain1/1 -> Sum/1
  Gain2/1 -> Derivative/1
  Derivative/1 -> Sum/3
  V/1 -> Add1/2, Gain2/1
  Vc/1 -> Gain1/1, Add1/1
  Add1/1 -> Gain/1
  thetac/1 -> Trigonometric Function1/1
  Trigonometric Function1/1 -> Product/2
  Sum/1 -> Product/1
  Product/1 -> LCV/1

== system Projet_Controle_Trajectoire_drone/Controle trajectoire1/U ==
  Xmes : Inport
  Ymes : Inport  Port=2
  Psic : Inport  Port=3
  Add : Sum
  Derivative : Derivative
  Derivative1 : Derivative
  Product : Product
  Product1 : Product
  Trigonometric Function : Trigonometry
  Trigonometric Function1 : Trigonometry  Operator=cos
  U : Outport
  wires:
  Trigonometric Function1/1 -> Product/2
  Product1/1 -> Add/2
  Product/1 -> Add/1
  Trigonometric Function/1 -> Product1/1
  Add/1 -> U/1
  Derivative1/1 -> Product1/2
  Psic/1 -> Trigonometric Function1/1, Trigonometric Function/1
  Xmes/1 -> Derivative/1
  Ymes/1 -> Derivative1/1
  Derivative/1 -> Product/1

== system Projet_Controle_Trajectoire_drone/Controle trajectoire1/Uc ==
  Xcorrigé : Inport
  Ycorrigé : Inport  Port=2
  Psic : Inport  Port=3
  Add : Sum
  Product : Product
  Product1 : Product
  Scope : Scope
  Trigonometric Function : Trigonometry
  Trigonometric Function1 : Trigonometry  Operator=cos
  Uc : Outport
  wires:
  Xcorrigé/1 -> Product/1, Scope/1
  Psic/1 -> Trigonometric Function1/1, Trigonometric Function/1
  Trigonometric Function1/1 -> Product/2
  Product/1 -> Add/1
  Trigonometric Function/1 -> Product1/1
  Ycorrigé/1 -> Product1/2
  Product1/1 -> Add/2
  Add/1 -> Uc/1

== system Projet_Controle_Trajectoire_drone/Controle trajectoire1/V ==
  Xmes : Inport
  Ymes : Inport  Port=2
  Psic : Inport  Port=3
  Add : Sum  Inputs=-+
  Derivative : Derivative
  Derivative1 : Derivative
  Product : Product
  Product1 : Product
  Trigonometric Function : Trigonometry  Operator=cos
  Trigonometric Function1 : Trigonometry
  V : Outport
  wires:
  Derivative/1 -> Product/1
  Derivative1/1 -> Product1/2
  Product1/1 -> Add/2
  Product/1 -> Add/1
  Xmes/1 -> Derivative/1
  Ymes/1 -> Derivative1/1
  Trigonometric Function1/1 -> Product/2
  Add/1 -> V/1
  Trigonometric Function/1 -> Product1/1
  Psic/1 -> Trigonometric Function1/1, Trigonometric Function/1

== system Projet_Controle_Trajectoire_drone/Controle trajectoire1/Vc ==
  Xcorrigé : Inport
  Ycorrigé : Inport  Port=2
  Psic : Inport  Port=3
  Add : Sum  Inputs=-+
  Product : Product
  Product1 : Product
  Trigonometric Function : Trigonometry  Operator=cos
  Trigonometric Function1 : Trigonometry
  Vc : Outport
  wires:
  Trigonometric Function/1 -> Product1/1
  Xcorrigé/1 -> Product/1
  Product1/1 -> Add/2
  Ycorrigé/1 -> Product1/2
  Add/1 -> Vc/1
  Trigonometric Function1/1 -> Product/2
  Product/1 -> Add/1
  Psic/1 -> Trigonometric Function/1, Trigonometric Function1/1

== system Projet_Controle_Trajectoire_drone/Quadrirotor/R ==
  note: Matrice de rotation du repère du drone vers le repère inertiel
  phi : Inport
  theta : Inport  Port=2
  psi : Inport  Port=3
  Matrix Multiply : Product  Inputs=***  Multiplication=Matrix(*)
  RotationX : Subsystem
  RotationY : Subsystem
  RotationZ : Subsystem
  R : Outport
  wires:
  phi/1 -> RotationX/1(angle)
  theta/1 -> RotationY/1(angle)
  psi/1 -> RotationZ/1(angle)
  Matrix Multiply/1 -> R/1
  RotationZ/1(Rz) -> Matrix Multiply/1
  RotationY/1(Ry) -> Matrix Multiply/2
  RotationX/1(Rx) -> Matrix Multiply/3

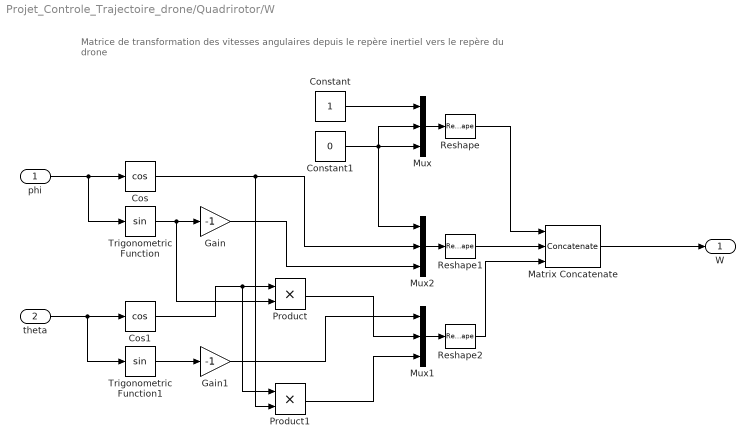
== system Projet_Controle_Trajectoire_drone/Quadrirotor/W ==
  note: Matrice de transformation des vitesses angulaires depuis le repère inertiel vers le repère du drone
  phi : Inport
  theta : Inport  Port=2
  Constant : Constant
  Constant1 : Constant  Value=0
  Cos : Trigonometry  Operator=cos
  Cos1 : Trigonometry  Operator=cos
  Gain : Gain  Gain=-1
  Gain1 : Gain  Gain=-1
  Matrix Concatenate : Concatenate  NumInputs=3  Mode=Multidimensional array  ConcatenateDimension=2
  Mux : Mux  Inputs=3
  Mux1 : Mux  Inputs=3
  Mux2 : Mux  Inputs=3
  Product : Product
  Product1 : Product
  Reshape : Reshape  OutputDimensionality=Column vector (2-D)
  Reshape1 : Reshape  OutputDimensionality=Column vector (2-D)
  Reshape2 : Reshape  OutputDimensionality=Column vector (2-D)
  Trigonometric Function : Trigonometry
  Trigonometric Function1 : Trigonometry
  W : Outport
  wires:
  Matrix Concatenate/1 -> W/1
  Product/1 -> Mux1/2
  Mux1/1 -> Reshape2/1
  Constant/1 -> Mux/1
  Mux2/1 -> Reshape1/1
  Constant1/1 -> Mux2/1, Mux/3, Mux/2
  Cos/1 -> Mux2/2, Product1/2
  phi/1 -> Cos/1, Trigonometric Function/1
  Gain/1 -> Mux2/3
  Trigonometric Function/1 -> Product/2, Gain/1
  Trigonometric Function1/1 -> Gain1/1
  theta/1 -> Trigonometric Function1/1, Cos1/1
  Gain1/1 -> Mux1/1
  Product1/1 -> Mux1/3
  Cos1/1 -> Product1/1, Product/1
  Mux/1 -> Reshape/1
  Reshape/1 -> Matrix Concatenate/1
  Reshape1/1 -> Matrix Concatenate/2
  Reshape2/1 -> Matrix Concatenate/3

== system Projet_Controle_Trajectoire_drone/Stabilisation/PID Phi ==
  e : Inport
  Derivative : Derivative
  Gain : Gain  Gain=KpPhi
  Gain1 : Gain  Gain=KiPhi
  Gain2 : Gain  Gain=KdPhi
  Integrator : Integrator
  Sum : Sum  Inputs=+|++
  u : Outport
  wires:
  Derivative/1 -> Sum/3
  Gain2/1 -> Derivative/1
  Integrator/1 -> Sum/1
  Gain1/1 -> Integrator/1
  Gain/1 -> Sum/2
  e/1 -> Gain/1, Gain1/1, Gain2/1
  Sum/1 -> u/1

== system Projet_Controle_Trajectoire_drone/Stabilisation/PID Psi ==
  e : Inport
  Derivative : Derivative
  Gain : Gain  Gain=KpPsi
  Gain1 : Gain  Gain=KiPsi
  Gain2 : Gain  Gain=KdPsi
  Integrator : Integrator
  Sum : Sum  Inputs=+|++
  u : Outport
  wires:
  Derivative/1 -> Sum/3
  Gain2/1 -> Derivative/1
  Integrator/1 -> Sum/1
  Gain1/1 -> Integrator/1
  Gain/1 -> Sum/2
  e/1 -> Gain/1, Gain1/1, Gain2/1
  Sum/1 -> u/1

== system Projet_Controle_Trajectoire_drone/Stabilisation/PID Theta ==
  e : Inport
  Derivative : Derivative
  Gain : Gain  Gain=KpTheta
  Gain1 : Gain  Gain=KiTheta
  Gain2 : Gain  Gain=KdTheta
  Integrator : Integrator
  Sum : Sum  Inputs=+|++
  u : Outport
  wires:
  Derivative/1 -> Sum/3
  Gain2/1 -> Derivative/1
  Integrator/1 -> Sum/1
  Gain1/1 -> Integrator/1
  Gain/1 -> Sum/2
  e/1 -> Gain/1, Gain1/1, Gain2/1
  Sum/1 -> u/1

== system Projet_Controle_Trajectoire_drone/Stabilisation/PID Z ==
  e : Inport
  Derivative : Derivative
  Gain : Gain  Gain=KpZ
  Gain1 : Gain  Gain=KiZ
  Gain2 : Gain  Gain=KdZ
  Integrator : Integrator
  Sum : Sum  Inputs=+|++
  u : Outport
  wires:
  Sum/1 -> u/1
  e/1 -> Gain2/1, Gain1/1, Gain/1
  Gain/1 -> Sum/2
  Gain1/1 -> Integrator/1
  Integrator/1 -> Sum/1
  Gain2/1 -> Derivative/1
  Derivative/1 -> Sum/3

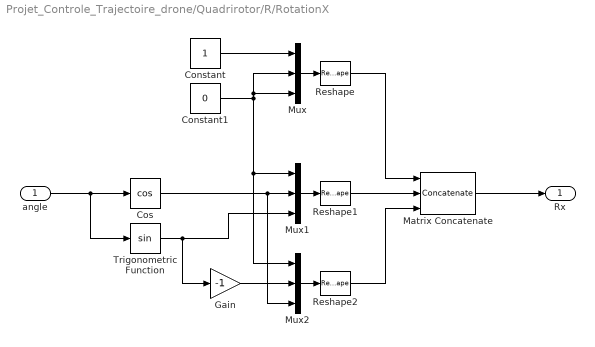
== system Projet_Controle_Trajectoire_drone/Quadrirotor/R/RotationX ==
  angle : Inport
  Constant : Constant
  Constant1 : Constant  Value=0
  Cos : Trigonometry  Operator=cos
  Gain : Gain  Gain=-1
  Matrix Concatenate : Concatenate  NumInputs=3  Mode=Multidimensional array  ConcatenateDimension=2
  Mux : Mux  Inputs=3
  Mux1 : Mux  Inputs=3
  Mux2 : Mux  Inputs=3
  Reshape : Reshape  OutputDimensionality=Column vector (2-D)
  Reshape1 : Reshape  OutputDimensionality=Column vector (2-D)
  Reshape2 : Reshape  OutputDimensionality=Column vector (2-D)
  Trigonometric Function : Trigonometry
  Rx : Outport
  wires:
  angle/1 -> Trigonometric Function/1, Cos/1
  Constant/1 -> Mux/1
  Constant1/1 -> Mux/3, Mux/2, Mux1/1, Mux2/1
  Cos/1 -> Mux2/3, Mux1/2
  Trigonometric Function/1 -> Mux1/3, Gain/1
  Gain/1 -> Mux2/2
  Matrix Concatenate/1 -> Rx/1
  Mux/1 -> Reshape/1
  Reshape/1 -> Matrix Concatenate/1
  Mux1/1 -> Reshape1/1
  Reshape1/1 -> Matrix Concatenate/2
  Mux2/1 -> Reshape2/1
  Reshape2/1 -> Matrix Concatenate/3

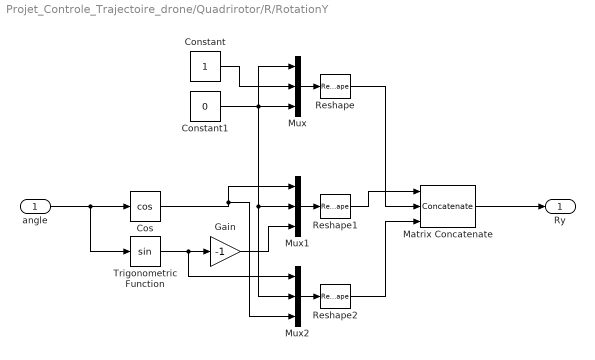
== system Projet_Controle_Trajectoire_drone/Quadrirotor/R/RotationY ==
  angle : Inport
  Constant : Constant
  Constant1 : Constant  Value=0
  Cos : Trigonometry  Operator=cos
  Gain : Gain  Gain=-1
  Matrix Concatenate : Concatenate  NumInputs=3  Mode=Multidimensional array  ConcatenateDimension=2
  Mux : Mux  Inputs=3
  Mux1 : Mux  Inputs=3
  Mux2 : Mux  Inputs=3
  Reshape : Reshape  OutputDimensionality=Column vector (2-D)
  Reshape1 : Reshape  OutputDimensionality=Column vector (2-D)
  Reshape2 : Reshape  OutputDimensionality=Column vector (2-D)
  Trigonometric Function : Trigonometry
  Ry : Outport
  wires:
  Matrix Concatenate/1 -> Ry/1
  Trigonometric Function/1 -> Mux2/1, Gain/1
  angle/1 -> Cos/1, Trigonometric Function/1
  Constant1/1 -> Mux/3, Mux/1, Mux2/2, Mux1/2
  Constant/1 -> Mux/2
  Cos/1 -> Mux2/3, Mux1/1
  Gain/1 -> Mux1/3
  Mux/1 -> Reshape/1
  Reshape/1 -> Matrix Concatenate/2
  Mux1/1 -> Reshape1/1
  Reshape1/1 -> Matrix Concatenate/1
  Mux2/1 -> Reshape2/1
  Reshape2/1 -> Matrix Concatenate/3

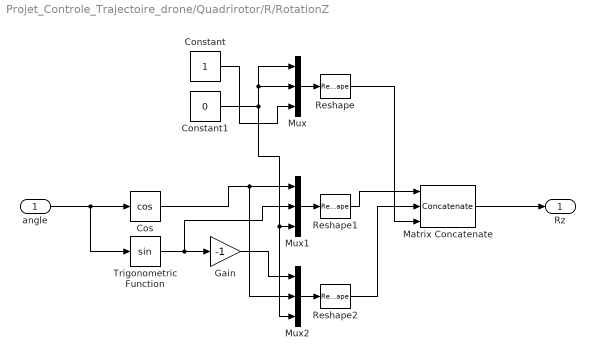
== system Projet_Controle_Trajectoire_drone/Quadrirotor/R/RotationZ ==
  angle : Inport
  Constant : Constant
  Constant1 : Constant  Value=0
  Cos : Trigonometry  Operator=cos
  Gain : Gain  Gain=-1
  Matrix Concatenate : Concatenate  NumInputs=3  Mode=Multidimensional array  ConcatenateDimension=2
  Mux : Mux  Inputs=3
  Mux1 : Mux  Inputs=3
  Mux2 : Mux  Inputs=3
  Reshape : Reshape  OutputDimensionality=Column vector (2-D)
  Reshape1 : Reshape  OutputDimensionality=Column vector (2-D)
  Reshape2 : Reshape  OutputDimensionality=Column vector (2-D)
  Trigonometric Function : Trigonometry
  Rz : Outport
  wires:
  angle/1 -> Trigonometric Function/1, Cos/1
  Trigonometric Function/1 -> Mux1/2, Gain/1
  Matrix Concatenate/1 -> Rz/1
  Constant1/1 -> Mux2/3, Mux1/3, Mux/1, Mux/2
  Constant/1 -> Mux/3
  Cos/1 -> Mux2/2, Mux1/1
  Gain/1 -> Mux2/1
  Mux/1 -> Reshape/1
  Reshape/1 -> Matrix Concatenate/3
  Mux1/1 -> Reshape1/1
  Reshape1/1 -> Matrix Concatenate/1
  Mux2/1 -> Reshape2/1
  Reshape2/1 -> Matrix Concatenate/2
